simulink model "Feedforward_parlante_mic_realtime"  (R2021b)
settings: Solver=FixedStepDiscrete  StartTime=0.0  StopTime=5.0  FixedStep=256/Fs  RelTol=1e-3
PreLoadFcn:
  | Fs = 44100;
  | f_tono = 500;
  | L = 32;
InitFcn:
  | Fs = 44100;
  | f_tono = 500;
  | L = 32;
undefined symbols (not defined in the file): SzEstimado
libraries: hdlsllib x3, audiosources x1, dspsnks4 x1, sldrtlib x1
settings Model: Creator=Vale Oieni  LastModifiedBy=ValeOieni

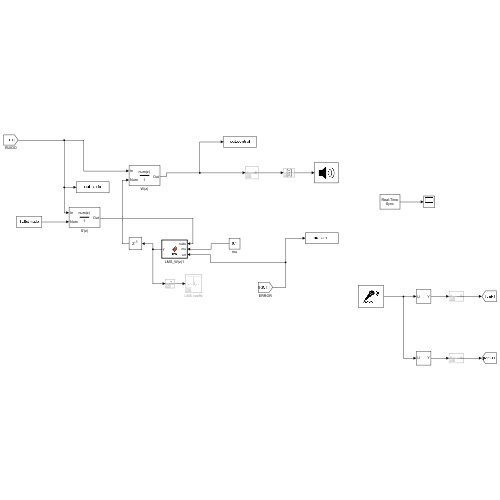
[thumbnail: Simulink's stored preview of the top-level diagram]
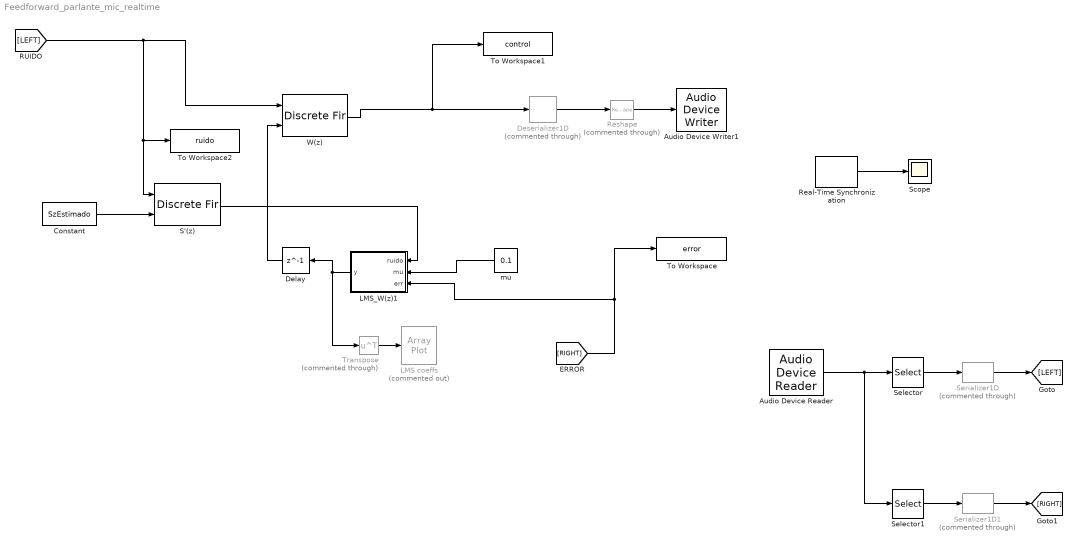
== system Feedforward_parlante_mic_realtime ==
  Audio Device Reader : audiosources/Audio Device Reader  Driver=ASIO  Device=ASIO4ALL v2  SampleRate=44100  NumChannels=2  SamplesPerFrame=256  BitDepth=16-bit integer  NumBuffers=10  DefaultInputChannelMapping=on  InputChannelMapping=1:2  OutputNumOverrunSamples=off  OutputDataType=double  DriverIdx=3  DeviceWarnFlag=''
      settings: SourceProductBaseCode=AU
  Audio Device Writer1 : dspsnks4/Audio Device Writer  Driver=ASIO  Device=ASIO4ALL v2  InheritSampleRate=off  SampleRate=44100  BitDepth=16-bit integer  BufferSize=4096  NumBuffers=10  DefaultOutputChannelMapping=on  OutputChannelMapping=1:2  OutputNumUnderrunSamples=off  DriverIdx=3  DeviceWarnFlag=''
  Constant : Constant  Value=SzEstimado  SampleTime=256/Fs
  Delay : Delay  DelayLength=1  InitialCondition=0  SampleTime=256/Fs
  Deserializer1D : hdlsllib/HDL Operations/Deserializer1D  Commented=through  Ratio=256  IdleCycles=0  InitialCondition=0  startIn=off  validIn=off  validOut=off  inputDataDimensions=-1  inputSampleTime=-1  inputSignalType=auto
      settings: SourceProductBaseCode=SL
  LMS coeffs : ArrayPlot  Commented=on  WindowPosition=[834.000000,474.000000,710.000000,384.000000,]  AxesScaling=Manual  YLimits=[-0.624999,0.624999]  ShowLegend=on  DefaultConfigurationName=dsp.scopes.ArrayPlotBlockSpecification
  LMS_W(z)1 : MATLAB Function  TreatAsAtomicUnit=on
  Real-Time Synchronization : sldrtlib/Real-Time Synchronization  SampleTime=256/Fs  MaxMissedTicks=10000000  ShowMissedTicks=on  YieldWhenWaiting=on
  Reshape : Reshape  Commented=through  OutputDimensionality=Column vector (2-D)  OutputDimensions=[2,1]
  S'(z) : DiscreteFir  CoefSource=Input port  InputProcessing=Columns as channels (frame based)
      settings: InputPortMap=u0,u1
  Scope : Scope
  Selector : Selector  NumberOfDimensions=2  InputPortWidth=3  IndexOptions=Select all,Index vector (dialog)  Indices=[1 3],1  OutputSizes=1,1
  Selector1 : Selector  NumberOfDimensions=2  InputPortWidth=3  IndexOptions=Select all,Index vector (dialog)  Indices=[1 3],2  OutputSizes=1,1
  Serializer1D : hdlsllib/HDL Operations/Serializer1D  Commented=through  Ratio=256  IdleCycles=0  validIn=off  startOut=off  validOut=off  inputDataDimensions=-1  inputSampleTime=-1  inputSignalType=auto
      settings: SourceProductBaseCode=SL
  Serializer1D1 : hdlsllib/HDL Operations/Serializer1D  Commented=through  Ratio=256  IdleCycles=0  validIn=off  startOut=off  validOut=off  inputDataDimensions=-1  inputSampleTime=-1  inputSignalType=auto
      settings: SourceProductBaseCode=SL
  To Workspace : ToWorkspace  VariableName=error  SampleTime=-1
      settings: Save2DSignal=2-D array (concatenate along first dimension)
  To Workspace1 : ToWorkspace  VariableName=control  SampleTime=-1
      settings: Save2DSignal=2-D array (concatenate along first dimension)
  To Workspace2 : ToWorkspace  VariableName=ruido  SampleTime=-1
      settings: Save2DSignal=2-D array (concatenate along first dimension)
  Transpose : Math  Commented=through  Operator=transpose  SignedPower=on  SaturateOnIntegerOverflow=on
  W(z) : DiscreteFir  CoefSource=Input port  InputProcessing=Columns as channels (frame based)
      settings: InputPortMap=u0,u1
  mu : Constant  Value=0.1  SampleTime=256/Fs
  wires:
  [RIGHT] -> LMS_W(z)1/3(err), To Workspace/1
  [LEFT] -> S'(z)/1, To Workspace2/1, W(z)/1
  Constant/1 -> S'(z)/2
  S'(z)/1 -> LMS_W(z)1/1(ruido)
  mu/1 -> LMS_W(z)1/2(mu)
  Transpose/1 -> LMS coeffs/1
  LMS_W(z)1/1(y) -> Delay/1, Transpose/1
  Delay/1 -> W(z)/2
  Serializer1D/1 -> [LEFT]
  Serializer1D1/1 -> [RIGHT]
  Selector/1 -> Serializer1D/1
  Audio Device Reader/1 -> Selector1/1, Selector/1
  Selector1/1 -> Serializer1D1/1
  Deserializer1D/1 -> Reshape/1
  Reshape/1 -> Audio Device Writer1/1
  W(z)/1 -> To Workspace1/1, Deserializer1D/1
  Real-Time Synchronization/1 -> Scope/1

== matlab function Feedforward_parlante_mic_realtime/LMS_W(z)1 ==
  data: ruido input; mu input; y output; err input
function y = fcn(ruido, mu, err)
    L = 128;
    %Pesos w_n
    persistent w_n
    if isempty(w_n)
        w_n = zeros(1, L); % inicializa w en cero, largo L
    end
    %Vector de ruido
    persistent x
    if isempty(x)
        x = zeros(1, L); % inicializa x en cero, largo L
    end
    %Vaciado de x
    for i = 1:length(ruido)
        x(2:L) = x(1:L-1);
        x(1) = ruido(i);
        %Actualizacion
        xvar = x;
        w = w_n;
        w = w + mu*err(i)*xvar;   
        w_n = w;
    end
    
    %Asignación a la salida
    y = w;
end
